simulink model "simulation2_PI"  (R2025b)
settings: Solver=ode3  StartTime=0.0  StopTime=10  FixedStep=0.1  RelTol=1e-3  EnableMultiTasking=on
undefined symbols (not defined in the file): dspblkCoreblockFVToolHelper, gcbh
libraries: arduinolib x3, arduinosensorlib x1
settings Model: ExtModeTrigDuration=2  Creator=20106  LastModifiedBy=asus
settings SolverCC: AutoInsertRateTranBlk=on
settings OptimizationCC: EnhancedBackFolding=on  PassReuseOutputArgsThreshold=0.0  MaxStackSize=64  OptimizeBlockOrder=speed  DifferentSizesBufferReuse=on  OptimizationCustomize=off
settings DebuggingCC: ParameterTunabilityLossMsg=error
settings HardwareCC: ProdBitPerInt=16.0  ProdBitPerPointer=16.0  ProdBitPerSizeT=16.0  ProdBitPerPtrDiffT=16.0  ProdLargestAtomicFloat=None  ProdWordSize=8.0  ProdHWDeviceType=Atmel->AVR
settings SFSimCC: MATLABDynamicMemAlloc=off
settings RTWCC: SystemTargetFile=ert.tlc  HardwareBoard=Arduino Uno  TemplateMakefile=ert_default_tmf  Toolchain=Arduino AVR  BuildConfiguration=Faster Runs  Description=Embedded Coder
settings CodeAppCC: ForceParamTrailComments=on  OperatorAnnotations=on
settings ERTTargetCC: ExtModeTransport=3.0  ExtModeStaticAlloc=on  ExtModeAutomaticAllocSize=off  ExtModeStaticAllocSize=250.0  ExtModeMexFile=ext_xcp  ExtModeIntrfLevel=Level2 - Open  InlinedParameterPlacement=Hierarchical  ERTCustomFileBanners=off  SupportContinuousTime=on  SupportNonInlinedSFcns=on  RemoveResetFunc=off  SupportVariableSizeSignals=on  ModelStepFunctionPrototypeControlCompliant=off

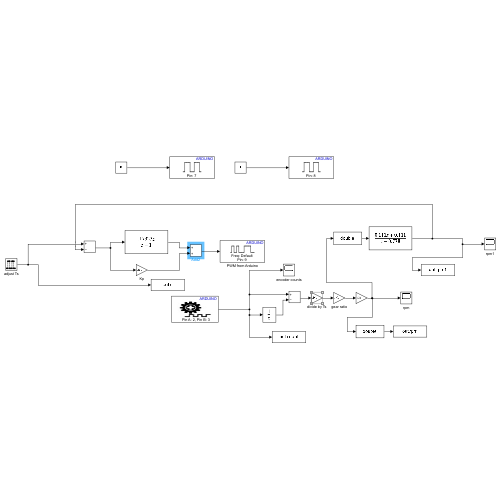
[thumbnail: Simulink's stored preview of the top-level diagram]
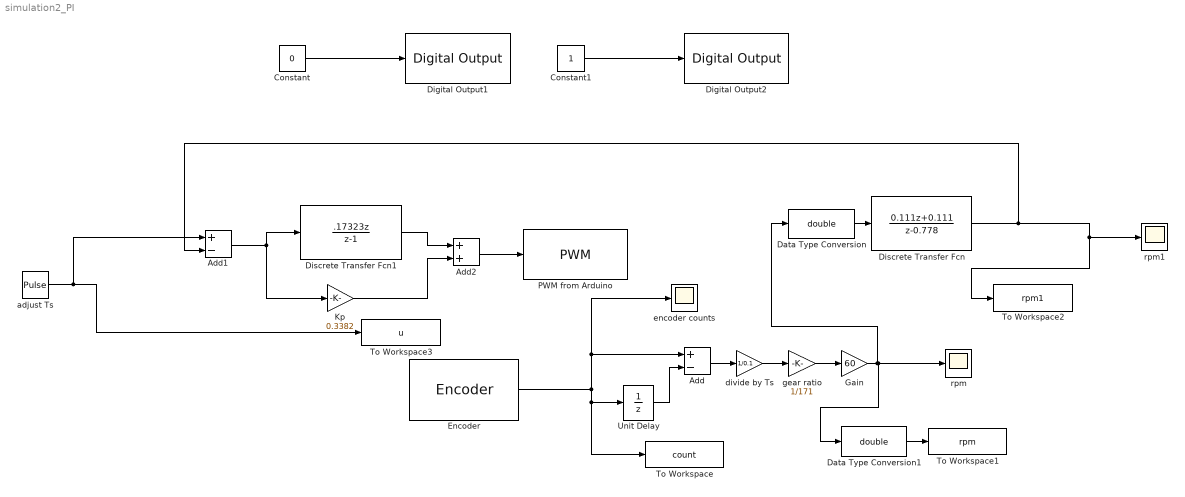
== system simulation2_PI ==
  Add : Sum  Inputs=+-
  Add1 : Sum  Inputs=+-
  Add2 : Sum
  Constant : Constant  Value=0
  Constant1 : Constant
  Data Type Conversion : DataTypeConversion  OutDataTypeStr=double  RndMeth=Nearest  SaturateOnIntegerOverflow=off
  Data Type Conversion1 : DataTypeConversion  OutDataTypeStr=double  RndMeth=Nearest  SaturateOnIntegerOverflow=off
  Digital Output1 : arduinolib/Digital Output  pinNumber=7  Direction=output  blockPlatform=arduino
  Digital Output2 : arduinolib/Digital Output  pinNumber=8  Direction=output  blockPlatform=arduino
  Discrete Transfer Fcn : DiscreteTransferFcn  LoadFcn=dspblkCoreblockFVToolHelper(gcbh,'load');  Numerator="[0.111  0.111]"  Denominator="[1   -0.778]"
      settings: CopyFcn=dspblkCoreblockFVToolHelper(gcbh,'copy');  DeleteFcn=dspblkCoreblockFVToolHelper(gcbh,'close');  ModelCloseFcn=dspblkCoreblockFVToolHelper(gcbh,'close');  PreSaveFcn=dspblkCoreblockFVToolHelper(gcbh,'presave');  PostSaveFcn=dspblkCoreblockFVToolHelper(gcbh,'postsave');  CloseFcn=dspblkCoreblockFVToolHelper(gcbh,'close');
  Discrete Transfer Fcn1 : DiscreteTransferFcn  LoadFcn=dspblkCoreblockFVToolHelper(gcbh,'load');  Numerator="[.17323  0]"  Denominator="[1   -1]"
      settings: CopyFcn=dspblkCoreblockFVToolHelper(gcbh,'copy');  DeleteFcn=dspblkCoreblockFVToolHelper(gcbh,'close');  ModelCloseFcn=dspblkCoreblockFVToolHelper(gcbh,'close');  PreSaveFcn=dspblkCoreblockFVToolHelper(gcbh,'presave');  PostSaveFcn=dspblkCoreblockFVToolHelper(gcbh,'postsave');  CloseFcn=dspblkCoreblockFVToolHelper(gcbh,'close');
  Encoder : arduinosensorlib/Encoder  InputA=2  InputB=3  Mode=Reset at each Sample time  SampleTime=.1
  Gain : Gain  Gain=60
  Kp : Gain  Gain=0.3382
  PWM from Arduino : arduinolib/PWM  pinNumber=9  frequencyType=Default  desiredFrequency=490.2  achievableFrequency=490.2
  To Workspace : ToWorkspace  VariableName=count  SaveFormat=Structure  SampleTime=-1
      settings: Save2DSignal=2-D array (concatenate along first dimension)
  To Workspace1 : ToWorkspace  VariableName=rpm  SampleTime=-1
      settings: Save2DSignal=2-D array (concatenate along first dimension)
  To Workspace2 : ToWorkspace  VariableName=rpm1  SampleTime=-1
      settings: Save2DSignal=2-D array (concatenate along first dimension)
  To Workspace3 : ToWorkspace  VariableName=u  SampleTime=-1
      settings: Save2DSignal=2-D array (concatenate along first dimension)
  Unit Delay : UnitDelay  SampleTime=-1  HasFrameUpgradeWarning=on
  "adjust Ts " : DiscretePulseGenerator  Period=150  PulseWidth=80  SampleTime=0.1
  divide by Ts : Gain  Gain=1/0.1
  encoder counts : Scope
      settings: ActiveDisplayYMinimum=-7799.125  ActiveDisplayYMaximum=70192.125
  gear ratio : Gain  Gain=1/171
  rpm : Scope
      settings: ActiveDisplayYMinimum=-13.25  ActiveDisplayYMaximum=119.25
  rpm1 : Scope
      settings: ActiveDisplayYMinimum=-4.87662  ActiveDisplayYMaximum=43.88956  DataLoggingVariableName=ScopeData2
  wires:
  "adjust Ts "/1 -> Add1/1, To Workspace3/1
  Constant/1 -> Digital Output1/1
  Constant1/1 -> Digital Output2/1
  Unit Delay/1 -> Add/2
  Encoder/1 -> To Workspace/1, Unit Delay/1, encoder counts/1, Add/1
  Add/1 -> divide by Ts/1
  divide by Ts/1 -> gear ratio/1
  gear ratio/1 -> Gain/1
  Gain/1 -> Data Type Conversion1/1, rpm/1, Data Type Conversion/1
  Data Type Conversion/1 -> Discrete Transfer Fcn/1
  Discrete Transfer Fcn/1 -> Add1/2, To Workspace2/1, rpm1/1
  Data Type Conversion1/1 -> To Workspace1/1
  Add1/1 -> Discrete Transfer Fcn1/1, Kp/1
  Discrete Transfer Fcn1/1 -> Add2/1
  Kp/1 -> Add2/2
  Add2/1 -> PWM from Arduino/1
